simulink model "Simulacion_posicion"  (R2015b)
settings: Solver=ode4  StartTime=0.0  StopTime=1.98  FixedStep=0.02  RelTol=1e-3
undefined symbols (not defined in the file): de_pos_cont, de_pos_disc, nu_pos_cont, nu_pos_disc
settings Model: Creator=sersanc8  LastModifiedBy=sersanc8

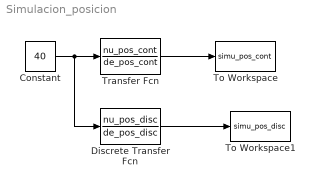
== system Simulacion_posicion ==
  Constant : Constant  Value=40
  Discrete Transfer Fcn : DiscreteTransferFcn  Numerator=nu_pos_disc  Denominator=de_pos_disc  SampleTime=0.02
  To Workspace : ToWorkspace  VariableName=simu_pos_cont  SampleTime=-1
  To Workspace1 : ToWorkspace  VariableName=simu_pos_disc  SampleTime=-1
  Transfer Fcn : TransferFcn  Numerator=nu_pos_cont  Denominator=de_pos_cont
  wires:
  Constant/1 -> Discrete Transfer Fcn/1, Transfer Fcn/1
  Transfer Fcn/1 -> To Workspace/1
  Discrete Transfer Fcn/1 -> To Workspace1/1
